simulink model "s0510_rollest_axleroll"  (R2021a)
settings: Solver=FixedStepAuto  StartTime=0.0  StopTime=10.0  FixedStep=0.001  RelTol=1e-3
libraries: CarMaker4SL x11
settings Model: Creator=jason  LastModifiedBy=jason

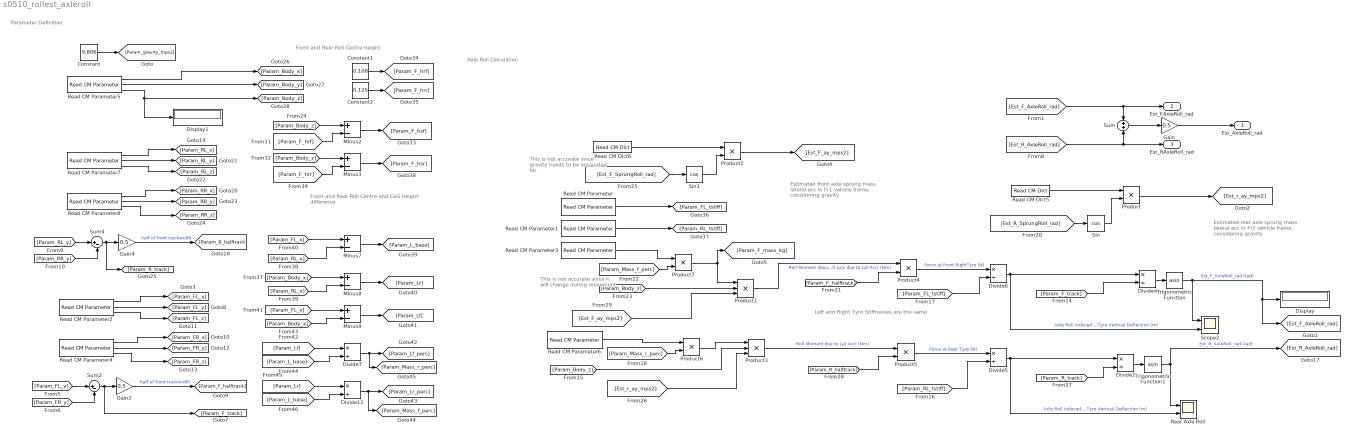
== system s0510_rollest_axleroll ==
  note: Front and Rear Roll Centre height
  note: Parameter Definition
  note: Axle Roll Calculation
  note: Left and Right Tyre Stiffnesses are the same
  note: Estimated front axle sprung mass lateral acc in Fr1 vehicle frame, considering gravity
  note: This is not accurate since it will change during movement
  note: This is not accurate since gravity needs to be accounted for
  note: Estimated rear axle sprung mass lateral acc in Fr1 vehicle frame, considering gravity
  note: Front and Rear Roll Centre and CoG height difference
  Constant : Constant  Value=9.806
  Constant1 : Constant  Value=0.108
  Constant2 : Constant  Value=0.125
  Display : Display
  Display1 : Display
  Divide{2,4..7,11} (6 alike) : Product  Inputs=*/
  Gain : Gain  Gain=0.5
  Gain2 : Gain  Gain=0.5
  Gain4 : Gain  Gain=0.5
  Minus{2..3,7..9} (5 alike) : Sum  Inputs=+-
  Product{,2,4..7} (6 alike) : Product
  Product1 : Product  Inputs=3
  Product3 : Product  Inputs=3
  Read CM Dict5 : CarMaker4SL/Read CM Dict  xname=Car.ay  xsync=off  xstime=Continuous
  Read CM Dict6 : CarMaker4SL/Read CM Dict  xname=Car.ay  xsync=off  xstime=Continuous
  Read CM Parameter : CarMaker4SL/Read CM Parameter  xfile=TireFL  xkey=Radial.Stiffness  xnout=1  xdefaults=0  xmuxed=on  xstime=Continuous
      settings: SourceProductName=CarMaker4SL
  Read CM Parameter1 : CarMaker4SL/Read CM Parameter  xfile=TireRL  xkey=Radial.Stiffness  xnout=1  xdefaults=0  xmuxed=on  xstime=Continuous
      settings: SourceProductName=CarMaker4SL
  Read CM Parameter2 : CarMaker4SL/Read CM Parameter  xfile=Vehicle  xkey=WheelCarrier.fl.pos  xnout=3  xdefaults=eps  xmuxed=off  xstime=Continuous
      settings: SourceProductName=CarMaker4SL
  Read CM Parameter3 : CarMaker4SL/Read CM Parameter  xfile=Vehicle  xkey=Body.mass  xnout=1  xdefaults=eps  xmuxed=off  xstime=Continuous
      settings: SourceProductName=CarMaker4SL
  Read CM Parameter4 : CarMaker4SL/Read CM Parameter  xfile=Vehicle  xkey=WheelCarrier.fr.pos  xnout=3  xdefaults=eps  xmuxed=off  xstime=Continuous
      settings: SourceProductName=CarMaker4SL
  Read CM Parameter5 : CarMaker4SL/Read CM Parameter  xfile=Vehicle  xkey=Body.pos  xnout=3  xdefaults=eps  xmuxed=off  xstime=Continuous
      settings: SourceProductName=CarMaker4SL
  Read CM Parameter6 : CarMaker4SL/Read CM Parameter  xfile=Vehicle  xkey=Body.mass  xnout=1  xdefaults=eps  xmuxed=off  xstime=Continuous
      settings: SourceProductName=CarMaker4SL
  Read CM Parameter7 : CarMaker4SL/Read CM Parameter  xfile=Vehicle  xkey=WheelCarrier.rl.pos  xnout=3  xdefaults=eps  xmuxed=off  xstime=Continuous
      settings: SourceProductName=CarMaker4SL
  Read CM Parameter8 : CarMaker4SL/Read CM Parameter  xfile=Vehicle  xkey=WheelCarrier.rr.pos  xnout=3  xdefaults=eps  xmuxed=off  xstime=Continuous
      settings: SourceProductName=CarMaker4SL
  Rear Axle Roll : Scope  NumInputPorts=2
  Scope2 : Scope  NumInputPorts=2
  Sin : Trigonometry  Operator=cos
  Sin1 : Trigonometry  Operator=cos
  Sum : Sum  Inputs=+|+
  Sum2 : Sum  Inputs=|+-
  Sum4 : Sum  Inputs=|+-
  Trigonometric Function : Trigonometry  Operator=asin
  Trigonometric Function1 : Trigonometry  Operator=asin
  Est_AxleRoll_rad : Outport
  Est_FAxleRoll_rad : Outport  Port=2
  Est_RAxleRoll_rad : Outport  Port=3
  wires:
  [Param_RR_y] -> Sum4/2
  Read CM Parameter3/1 -> Product7/1
  Sin/1 -> Product/2
  [Est_F_SprungRoll_rad] -> Sin1/1
  Read CM Parameter4/2 -> [Param_FR_y]
  [Est_r_ay_mps2] -> Product3/3
  [Est_F_ay_mps2] -> Product1/3
  Sin1/1 -> Product2/2
  Trigonometric Function1/1 -> Rear Axle Roll/1, [Est_R_AxleRoll_rad]  "Est_R_AxleRoll_rad (rad)"
  Read CM Parameter8/1 -> [Param_RR_x]
  Read CM Dict6/1 -> Product2/1
  Product/1 -> [Est_r_ay_mps2]
  Product3/1 -> Product5/1  "Roll Moment due to Lat Accl (Nm)"
  Product7/1 -> [Param_F_mass_kg], Product1/1
  Divide4/1 -> Trigonometric Function/1
  Product2/1 -> [Est_F_ay_mps2]
  Read CM Parameter2/3 -> [Param_FL_z]
  Read CM Parameter/1 -> [Param_FL_tstiff]
  Gain2/1 -> [Param_F_halftrack]  "half of front trackwidth"
  Read CM Parameter2/1 -> [Param_FL_x]
  [Param_FL_y] -> Sum2/1
  [Est_R_SprungRoll_rad] -> Sin/1
  Product6/1 -> Product3/1
  Constant/1 -> [Param_gravity_mps2]
  Product1/1 -> Product4/1  "Roll Moment about roll axis due to Lat Accl (Nm)"
  Sum4/1 -> Gain4/1, [Param_R_track]
  Divide6/1 -> Divide4/1, Scope2/2  "Axle Roll induced Tyre Vertical Deflection (m)"
  Read CM Parameter1/1 -> [Param_RL_tstiff]
  Read CM Parameter6/1 -> Product6/1
  [Param_F_track] -> Divide4/2
  [Param_F_halftrack] -> Product4/2
  Product4/1 -> Divide6/1  "Force at Front RightTyre (N)"
  [Param_Body_z] -> Product3/2
  Product5/1 -> Divide5/1  "Force at Rear Tyre (N)"
  Divide2/1 -> Trigonometric Function1/1
  [Param_FL_tstiff] -> Divide6/2
  [Param_R_track] -> Divide2/2
  Trigonometric Function/1 -> Scope2/1, [Est_F_AxleRoll_rad], Display/1  "Est_F_AxleRoll_rad (rad)"
  Sum2/1 -> Gain2/1, [Param_F_track]
  Read CM Parameter5/2 -> [Param_Body_y]
  [Param_RL_tstiff] -> Divide5/2
  [Param_Body_z] -> Product1/2
  Read CM Parameter5/1 -> [Param_Body_x]
  [Param_RL_y] -> Sum4/1
  Divide5/1 -> Divide2/1, Rear Axle Roll/2  "Axle Roll induced Tyre Vertical Deflection (m)"
  Read CM Parameter2/2 -> [Param_FL_y]
  Read CM Parameter5/3 -> Display1/1, [Param_Body_z]
  [Param_R_halftrack] -> Product5/2
  Gain4/1 -> [Param_R_halftrack]  "half of front trackwidth"
  [Param_FR_y] -> Sum2/2
  Read CM Parameter8/2 -> [Param_RR_y]
  Read CM Parameter4/3 -> [Param_FR_z]
  Read CM Parameter4/1 -> [Param_FR_x]
  Read CM Parameter7/1 -> [Param_RL_x]
  Read CM Parameter8/3 -> [Param_RR_z]
  Read CM Parameter7/3 -> [Param_RL_z]
  Read CM Parameter7/2 -> [Param_RL_y]
  Read CM Dict5/1 -> Product/1
  Constant1/1 -> [Param_F_hrf]
  Constant2/1 -> [Param_F_hrr]
  [Param_F_hrf] -> Minus2/2
  [Param_Body_z] -> Minus2/1
  Minus2/1 -> [Param_F_hsf]
  Minus3/1 -> [Param_F_hsr]
  [Param_Body_z] -> Minus3/1
  [Param_F_hrr] -> Minus3/2
  [Param_Body_x] -> Minus8/1
  [Param_RL_x] -> Minus7/2
  [Param_FL_x] -> Minus7/1
  Minus7/1 -> [Param_L_base]
  [Param_RL_x] -> Minus8/2
  Minus8/1 -> [Param_Lr]
  [Param_FL_x] -> Minus9/1
  [Param_Body_x] -> Minus9/2
  Minus9/1 -> [Param_Lf]
  [Param_Lf] -> Divide7/1
  [Param_L_base] -> Divide7/2
  Divide7/1 -> [Param_Mass_r_perc], [Param_Lf_perc]
  Divide11/1 -> [Param_Mass_f_perc], [Param_Lr_perc]
  [Param_L_base] -> Divide11/2
  [Param_Lr] -> Divide11/1
  [Param_Mass_f_perc] -> Product7/2
  [Param_Mass_r_perc] -> Product6/2
  [Est_F_AxleRoll_rad] -> Sum/1, Est_FAxleRoll_rad/1
  [Est_R_AxleRoll_rad] -> Sum/2, Est_RAxleRoll_rad/1
  Sum/1 -> Gain/1
  Gain/1 -> Est_AxleRoll_rad/1
